simulink model "Model2"  (R2017a)
settings: Solver=ode23t  StartTime=0.0  StopTime=10.0  RelTol=1e-4
values from neighbouring files (symbols this model uses):
  param = evalin('base','param')    [getSaveInfo.m]    (also in loadBackUp.m)
(part 1 of 3)
settings Model: Creator=www  LastModifiedBy=www
settings SolverCC: MaxConsecutiveMinStep=1000  ShapePreserveControl=EnableAll  ZeroCrossAlgorithm=Adaptive
settings DataIOCC: SaveOutput=off  SignalLogging=off  DSMLogging=off  SaveTime=off

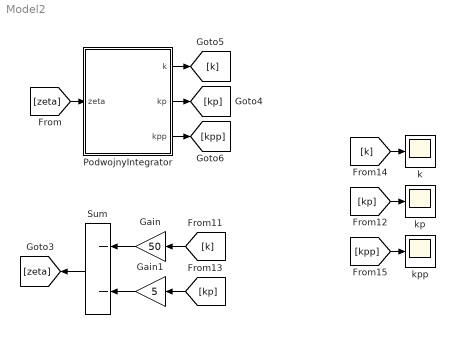
== system Model2 ==
  Gain : Gain  Gain=50
  Gain1 : Gain  Gain=5
  PodwojnyIntegrator : Subsystem
  Sum : Sum  Inputs=--
  k : Scope
  kp : Scope
  kpp : Scope
  wires:
  Sum/1 -> [zeta]
  Gain/1 -> Sum/1
  Gain1/1 -> Sum/2
  [k] -> Gain/1
  [kp] -> kp/1
  PodwojnyIntegrator/2(kp) -> [kp]
  PodwojnyIntegrator/1(k) -> [k]
  PodwojnyIntegrator/3(kpp) -> [kpp]
  [kp] -> Gain1/1
  [k] -> k/1
  [kpp] -> kpp/1
  [zeta] -> PodwojnyIntegrator/1(zeta)

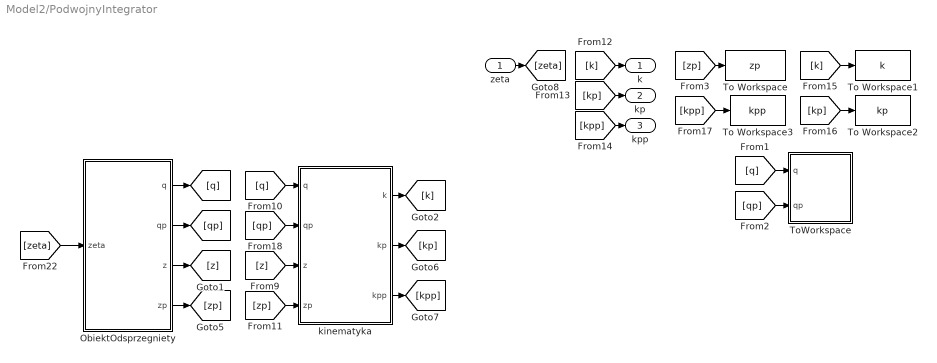
== system Model2/PodwojnyIntegrator ==
  zeta : Inport
  ObiektOdsprzegniety : Subsystem
  To Workspace : ToWorkspace  VariableName=zp  SaveFormat=Timeseries  SampleTime=-1
  To Workspace1 : ToWorkspace  VariableName=k  SaveFormat=Timeseries  SampleTime=-1
  To Workspace2 : ToWorkspace  VariableName=kp  SaveFormat=Timeseries  SampleTime=-1
  To Workspace3 : ToWorkspace  VariableName=kpp  SaveFormat=Timeseries  SampleTime=-1
  "ToWorkspace " : Subsystem
  kinematyka : MATLAB Function  TreatAsAtomicUnit=on
  k : Outport
  kp : Outport  Port=2
  kpp : Outport  Port=3
  wires:
  [zp] -> To Workspace/1
  [z] -> kinematyka/3(z)
  [q] -> kinematyka/1(q)
  [zp] -> kinematyka/4(zp)
  [k] -> k/1
  [kp] -> kp/1
  [kpp] -> kpp/1
  kinematyka/1(k) -> [k]
  kinematyka/2(kp) -> [kp]
  kinematyka/3(kpp) -> [kpp]
  [k] -> To Workspace1/1
  [kp] -> To Workspace2/1
  [kpp] -> To Workspace3/1
  [qp] -> kinematyka/2(qp)
  zeta/1 -> [zeta]
  [zeta] -> ObiektOdsprzegniety/1(zeta)
  ObiektOdsprzegniety/3(z) -> [z]
  ObiektOdsprzegniety/4(zp) -> [zp]
  [qp] -> "ToWorkspace "/2(qp)
  [q] -> "ToWorkspace "/1(q)
  ObiektOdsprzegniety/2(qp) -> [qp]
  ObiektOdsprzegniety/1(q) -> [q]

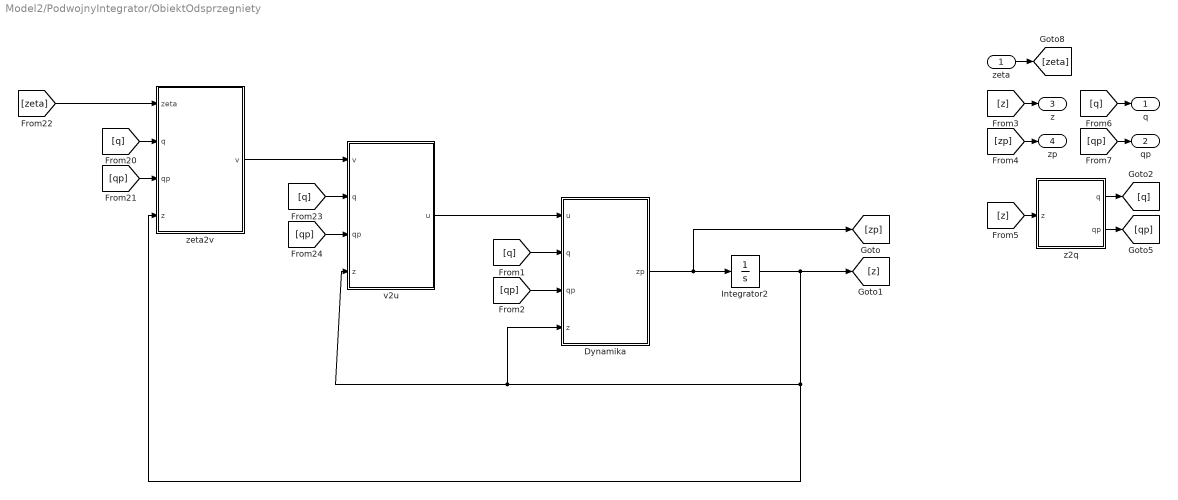
== system Model2/PodwojnyIntegrator/ObiektOdsprzegniety ==
  zeta : Inport
  Dynamika : MATLAB Function  TreatAsAtomicUnit=on
  Integrator2 : Integrator  InitialCondition=param.initCond.z0
  v2u : MATLAB Function  TreatAsAtomicUnit=on
  z2q : Subsystem
  zeta2v : MATLAB Function  TreatAsAtomicUnit=on
  q : Outport
  qp : Outport  Port=2
  z : Outport  Port=3
  zp : Outport  Port=4
  wires:
  [q] -> zeta2v/2(q)
  [qp] -> v2u/3(qp)
  zeta2v/1(v) -> v2u/1(v)
  [qp] -> zeta2v/3(qp)
  [q] -> v2u/2(q)
  [zeta] -> zeta2v/1(zeta)
  zeta/1 -> [zeta]
  Dynamika/1(zp) -> Integrator2/1, [zp]
  v2u/1(u) -> Dynamika/1(u)
  [qp] -> Dynamika/3(qp)
  [q] -> Dynamika/2(q)
  [z] -> z/1
  [zp] -> zp/1
  Integrator2/1 -> zeta2v/4(z), v2u/4(z), Dynamika/4(z), [z]
  [z] -> z2q/1(z)
  z2q/1(q) -> [q]
  z2q/2(qp) -> [qp]
  [qp] -> qp/1
  [q] -> q/1

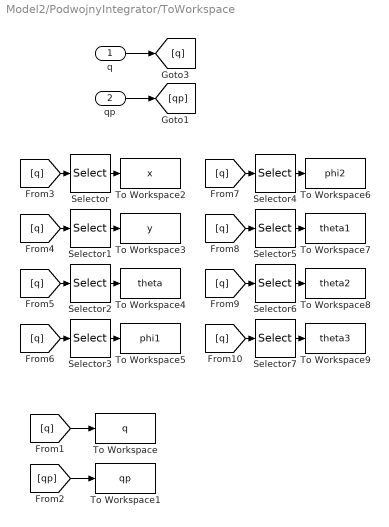
== system Model2/PodwojnyIntegrator/ToWorkspace  ==
  q : Inport
  qp : Inport  Port=2
  Selector : Selector  InputPortWidth=8  IndexOptions=Index vector (dialog)  Indices=1  OutputSizes=1
  Selector1 : Selector  InputPortWidth=8  IndexOptions=Index vector (dialog)  Indices=2  OutputSizes=1
  Selector2 : Selector  InputPortWidth=8  IndexOptions=Index vector (dialog)  Indices=3  OutputSizes=1
  Selector3 : Selector  InputPortWidth=8  IndexOptions=Index vector (dialog)  Indices=4  OutputSizes=1
  Selector4 : Selector  InputPortWidth=8  IndexOptions=Index vector (dialog)  Indices=5  OutputSizes=1
  Selector5 : Selector  InputPortWidth=8  IndexOptions=Index vector (dialog)  Indices=6  OutputSizes=1
  Selector6 : Selector  InputPortWidth=8  IndexOptions=Index vector (dialog)  Indices=7  OutputSizes=1
  Selector7 : Selector  InputPortWidth=8  IndexOptions=Index vector (dialog)  Indices=8  OutputSizes=1
  To Workspace : ToWorkspace  VariableName=q  SaveFormat=Timeseries  SampleTime=-1
  To Workspace1 : ToWorkspace  VariableName=qp  SaveFormat=Timeseries  SampleTime=-1
  To Workspace2 : ToWorkspace  VariableName=x  SampleTime=-1
  To Workspace3 : ToWorkspace  VariableName=y  SampleTime=-1
  To Workspace4 : ToWorkspace  VariableName=theta  SaveFormat=Timeseries  SampleTime=-1
  To Workspace5 : ToWorkspace  VariableName=phi1  SaveFormat=Timeseries  SampleTime=-1
  To Workspace6 : ToWorkspace  VariableName=phi2  SaveFormat=Timeseries  SampleTime=-1
  To Workspace7 : ToWorkspace  VariableName=theta1  SaveFormat=Timeseries  SampleTime=-1
  To Workspace8 : ToWorkspace  VariableName=theta2  SaveFormat=Timeseries  SampleTime=-1
  To Workspace9 : ToWorkspace  VariableName=theta3  SaveFormat=Timeseries  SampleTime=-1
  wires:
  Selector/1 -> To Workspace2/1
  [q] -> Selector/1
  Selector1/1 -> To Workspace3/1
  [q] -> Selector1/1
  Selector2/1 -> To Workspace4/1
  [q] -> Selector2/1
  Selector3/1 -> To Workspace5/1
  [q] -> Selector3/1
  Selector4/1 -> To Workspace6/1
  [q] -> Selector4/1
  Selector5/1 -> To Workspace7/1
  [q] -> Selector5/1
  Selector6/1 -> To Workspace8/1
  [q] -> Selector6/1
  Selector7/1 -> To Workspace9/1
  [q] -> Selector7/1
  [qp] -> To Workspace1/1
  [q] -> To Workspace/1
  q/1 -> [q]
  qp/1 -> [qp]

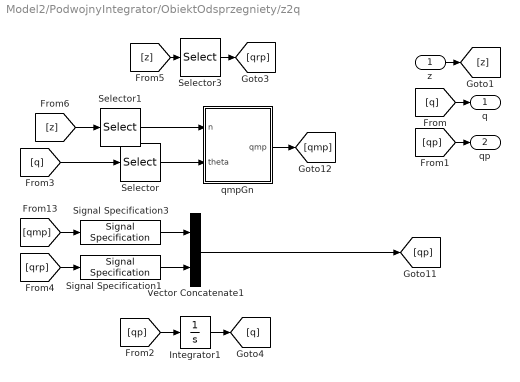
== system Model2/PodwojnyIntegrator/ObiektOdsprzegniety/z2q ==
  z : Inport
  Integrator1 : Integrator  InitialCondition=[param.initCond.qm0,param.initCond.qr0]
  Selector : Selector  InputPortWidth=8  IndexOptions=Index vector (dialog)  Indices=[3]  OutputSizes=1
  Selector1 : Selector  InputPortWidth=5  IndexOptions=Index vector (dialog)  Indices=[1 2]  OutputSizes=1
  Selector3 : Selector  InputPortWidth=5  IndexOptions=Index vector (dialog)  Indices=[3 4 5]  OutputSizes=1
  Signal Specification1 : SignalSpecification  Dimensions=[1 3]
  Signal Specification3 : SignalSpecification  Dimensions=[1 5]
  Vector Concatenate1 : Concatenate
  qmpGn : MATLAB Function  TreatAsAtomicUnit=on
  q : Outport
  qp : Outport  Port=2
  wires:
  z/1 -> [z]
  [q] -> q/1
  [qp] -> qp/1
  [z] -> Selector1/1
  Selector/1 -> qmpGn/2(theta)
  [qmp] -> Signal Specification3/1
  [qrp] -> Signal Specification1/1
  Selector3/1 -> [qrp]
  [z] -> Selector3/1
  [qp] -> Integrator1/1
  Integrator1/1 -> [q]
  [q] -> Selector/1
  Selector1/1 -> qmpGn/1(n)
  qmpGn/1(qmp) -> [qmp]
  Signal Specification3/1 -> Vector Concatenate1/1
  Signal Specification1/1 -> Vector Concatenate1/2
  Vector Concatenate1/1 -> [qp]

== matlab function Model2/PodwojnyIntegrator/ObiektOdsprzegniety/z2q/qmpGn ==
  data: n input; qmp output; theta input
function qmp = fcn(n,theta)
L=0.3;
R=0.075;
qmp=[cos(theta), cos(theta);
    sin(theta), sin(theta)
    1/L, -1/L;
    2/R, 0;
    0, 2/R]*n;
